simulink model "Model"  (R2018a)
settings: Solver=ode2  StartTime=0.0  StopTime=inf  FixedStep=Ts  RelTol=1e-3
PreLoadFcn:
  | k_synchronize=2;
InitFcn:
  | k_synchronize=2;
  | lego_drive_closedloop_InitData.mdl = get_param(bdroot,'Name');
  | lego_drive_closedloop_InitData.cs = getActiveConfigSet(lego_drive_closedloop_InitData.mdl);
values from neighbouring files (symbols this model uses):
  AxeLength = 31    [robotParam.m]
  D_DeadBand = 2    [robotParam.m]
  EncRes = 2048    [robotParam.m]
  RateLimitHigh = 10    [robotParam.m]
  RateLimitLow = -30    [robotParam.m]
  theta0 = 0    [robotParam.m]
  WheelRadius = 2    [robotParam.m]
  x0 = 0    [robotParam.m]
  y0 = 0    [robotParam.m]
libraries: arduinolib x6, simulink x3, simulink_extras x1
CloseFcn:
  | clear k_synchronize lego_drive_closedloop_InitData
settings Model: SimulationMode=external  ExtModeTrigDuration=2  Creator=The MathWorks, Inc.  LastModifiedBy=root
settings DataIOCC: LimitDataPoints=on  SaveFormat=Array
settings OptimizationCC: ExpressionDepthLimit=2147483647  LifeSpan=Inf  MaxStackSize=64
settings DebuggingCC: UnderspecifiedInitializationDetection=Classic  MergeDetectMultiDrivingBlocksExec=none  InheritedTsInSrcMsg=none  ParameterPrecisionLossMsg=none  FcnCallInpInsideContextMsg=warning  AllowSymbolicDim=off  StateNameClashWarn=warning  SFUnexpectedBacktrackingDiag=warning  SFNoUnconditionalDefaultTransitionDiag=warning  SFExecutionAtInitializationDiag=none
settings HardwareCC: ProdBitPerInt=16  ProdBitPerPointer=16  ProdBitPerSizeT=16  ProdBitPerPtrDiffT=16  ProdLargestAtomicFloat=None  ProdWordSize=8  ProdHWDeviceType=Atmel->AVR  UseEmbeddedCoderFeatures=off  UseSimulinkCoderFeatures=off
settings ModelReferenceCC: PropagateSignalLabelsOutOfModel=off
settings SFSimCC: MATLABDynamicMemAlloc=off
settings RTWCC: SystemTargetFile=ert.tlc  HardwareBoard=Arduino Mega 2560  TemplateMakefile=ert_default_tmf  GenerateReport=on  RTWVerbose=off  Toolchain=Arduino AVR  BuildConfiguration=Faster Runs  LaunchReport=on
settings CodeAppCC: ForceParamTrailComments=on  OperatorAnnotations=on  MangleLength=10  StateflowObjectComments=on  MATLABSourceComments=on
settings ERTTargetCC: MultiwordLength=2048  ERTCustomFileBanners=off  SupportContinuousTime=on  SupportNonInlinedSFcns=on  RemoveResetFunc=off  ModelStepFunctionPrototypeControlCompliant=off
settings ConfigComp: CovMetricSettings=dw  CovHtmlReporting=on  CovSaveCumulativeToWorkspaceVar=on  CovSaveSingleToWorkspaceVar=on  CovExternalEMLEnable=off  CovSFcnEnable=off

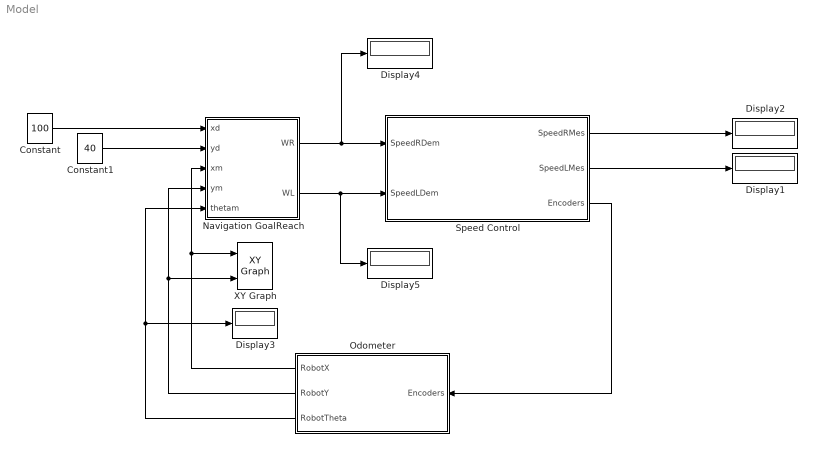
== system Model ==
  Constant : Constant  Value=100
  Constant1 : Constant  Value=40
  Display{1..5} (5 alike) : Display
  Navigation GoalReach : Subsystem
  Odometer : Subsystem
  Speed Control : Subsystem
  XY Graph : simulink/Sinks/XY Graph  xmin=-50  xmax=120  ymin=-50  ymax=120  st=-1
  wires:
  Navigation GoalReach/1(WR) -> Display4/1, Speed Control/1(SpeedRDem)
  Navigation GoalReach/2(WL) -> Display5/1, Speed Control/2(SpeedLDem)
  Speed Control/2(SpeedLMes) -> Display1/1
  Odometer/1(RobotX) -> XY Graph/1, Navigation GoalReach/3(xm)
  Odometer/2(RobotY) -> XY Graph/2, Navigation GoalReach/4(ym)
  Odometer/3(RobotTheta) -> Display3/1, Navigation GoalReach/5(thetam)
  Constant/1 -> Navigation GoalReach/1(xd)
  Constant1/1 -> Navigation GoalReach/2(yd)
  Speed Control/1(SpeedRMes) -> Display2/1
  Speed Control/3(Encoders) -> Odometer/1(Encoders)

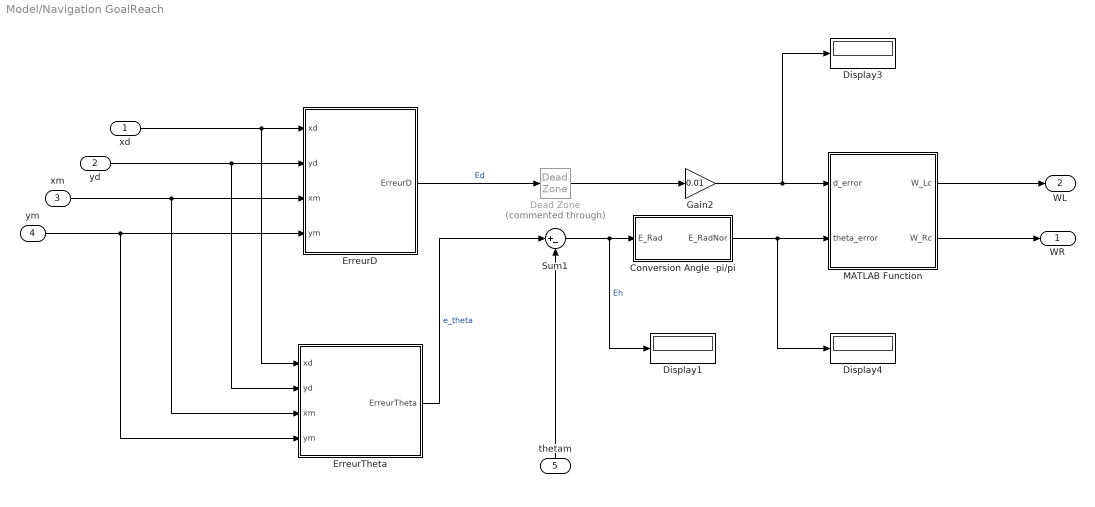
== system Model/Navigation GoalReach ==
  xd : Inport
  yd : Inport  Port=2
  xm : Inport  Port=3
  ym : Inport  Port=4
  thetam : Inport  Port=5
  Conversion Angle -pi/pi : Subsystem
  Dead Zone : DeadZone  Commented=through  LowerValue=-D_DeadBand  UpperValue=D_DeadBand  SaturateOnIntegerOverflow=on
  Display1 : Display
  Display3 : Display
  Display4 : Display
  ErreurD : Subsystem
  ErreurTheta : Subsystem
  Gain2 : Gain  Gain=0.01
  MATLAB Function : MATLAB Function  TreatAsAtomicUnit=on
  Sum1 : Sum  Inputs=|+-
  WR : Outport
  WL : Outport  Port=2
  wires:
  ErreurTheta/1(ErreurTheta) -> Sum1/1  "e_theta"
  xm/1 -> ErreurTheta/3(xm), ErreurD/3(xm)
  ym/1 -> ErreurTheta/4(ym), ErreurD/4("ym ")
  ErreurD/1(ErreurD) -> Dead Zone/1  "Ed"
  Sum1/1 -> Conversion Angle -pi/pi/1("E_Rad "), Display1/1  "Eh"
  thetam/1 -> Sum1/2
  xd/1 -> ErreurTheta/1(xd), ErreurD/1(xd)
  yd/1 -> ErreurTheta/2(yd), ErreurD/2(yd)
  Gain2/1 -> Display3/1, MATLAB Function/1(d_error)
  Conversion Angle -pi/pi/1(E_RadNor) -> Display4/1, MATLAB Function/2(theta_error)
  Dead Zone/1 -> Gain2/1
  MATLAB Function/1(W_Lc) -> WL/1
  MATLAB Function/2(W_Rc) -> WR/1

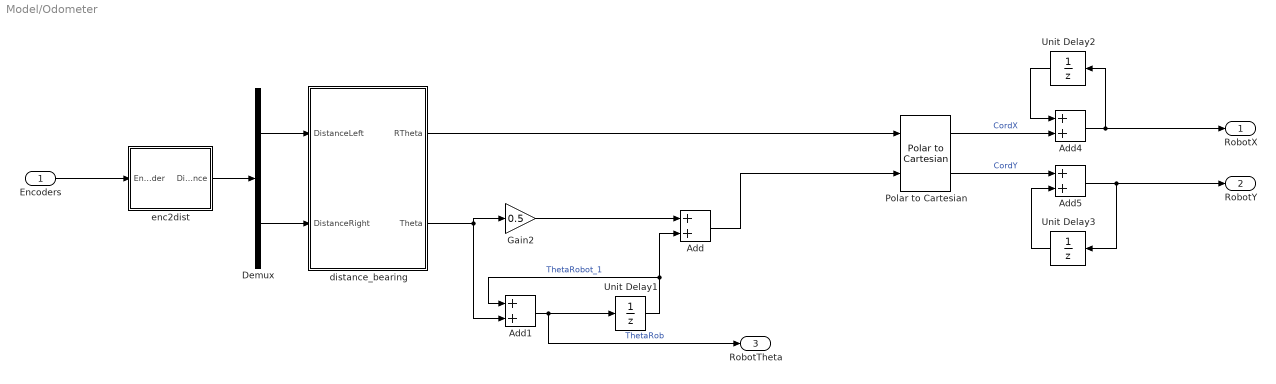
== system Model/Odometer ==
  Encoders : Inport
  Add{,1,4..5} (4 alike) : Sum
  Demux : Demux  Outputs=2
  Gain2 : Gain  Gain=0.5
  Polar to Cartesian : simulink_extras/Transformations/Polar to Cartesian
      settings: SourceProductName=Simulink  SourceProductBaseCode=SL
  Unit Delay1 : UnitDelay  DialogController=Simulink.DDGSource  InitialCondition=theta0*pi/180  SampleTime=-1
  Unit Delay2 : UnitDelay  DialogController=Simulink.DDGSource  InitialCondition=x0  SampleTime=-1
  Unit Delay3 : UnitDelay  DialogController=Simulink.DDGSource  InitialCondition=y0  SampleTime=-1
  distance_bearing : Subsystem
  enc2dist : Subsystem
  RobotX : Outport
  RobotY : Outport  Port=2
  RobotTheta : Outport  Port=3
  wires:
  Gain2/1 -> Add/1
  Polar to Cartesian/1 -> Add4/2  "CordX"
  Polar to Cartesian/2 -> Add5/1  "CordY"
  Unit Delay2/1 -> Add4/1
  Unit Delay3/1 -> Add5/2
  distance_bearing/2(Theta) -> Gain2/1, Add1/2
  Unit Delay1/1 -> Add1/1, Add/2  "ThetaRobot_1"
  Add/1 -> Polar to Cartesian/2
  Add1/1 -> RobotTheta/1, Unit Delay1/1  "ThetaRob"
  distance_bearing/1(RTheta) -> Polar to Cartesian/1
  Add4/1 -> RobotX/1, Unit Delay2/1
  enc2dist/1(Distance) -> Demux/1
  Demux/1 -> distance_bearing/1(DistanceLeft)
  Demux/2 -> distance_bearing/2(DistanceRight)
  Encoders/1 -> enc2dist/1(Encoder)
  Add5/1 -> RobotY/1, Unit Delay3/1

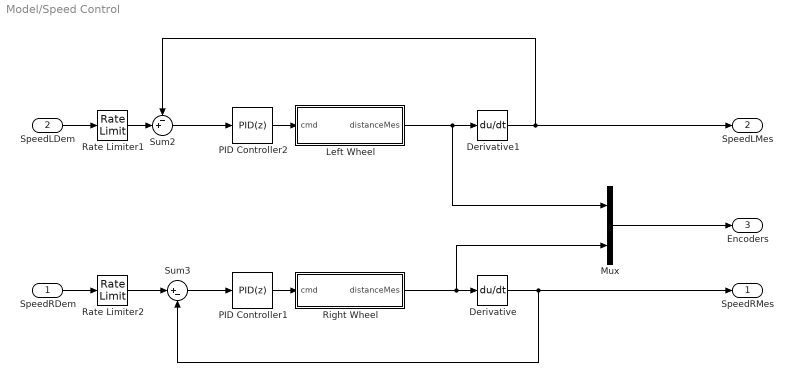
== system Model/Speed Control ==
  SpeedRDem : Inport
  SpeedLDem : Inport  Port=2
  " Left Wheel" : Subsystem
  Derivative : Derivative
  Derivative1 : Derivative
  Mux : Mux  Inputs=2
  PID Controller1 : simulink/Continuous/PID Controller  Controller=PID  TimeDomain=Discrete-time  SampleTime=-1  IntegratorMethod=Forward Euler  FilterMethod=Forward Euler  Form=Parallel  UseFilter=off  ControllerParametersSource=internal  P=0.030  I=0.001  D=0  N=1  InitialConditionSource=internal  InitialConditionForIntegrator=0  InitialConditionForFilter=0  ExternalReset=none  LimitOutput=on  UpperSaturationLimit=1  LowerSaturationLimit=-1  LinearizeAsGain=on  AntiWindupMode=clamping  Kb=1  TrackingMode=off  Kt=1  PParamMin=[]  PParamMax=[]  IParamMin=[]  IParamMax=[]  DParamMin=[]  DParamMax=[]  NParamMin=[]  NParamMax=[]  KbParamMin=[]  KbParamMax=[]  KtParamMin=[]  KtParamMax=[]  POutMin=[]  POutMax=[]  IOutMin=[]  IOutMax=[]  DOutMin=[]  DOutMax=[]  NOutMin=[]  NOutMax=[]  KbOutMin=[]  KbOutMax=[]  KtOutMin=[]  KtOutMax=[]  IntegratorOutMin=[]  IntegratorOutMax=[]  FilterOutMin=[]  FilterOutMax=[]  SumOutMin=[]  SumOutMax=[]  SumI1OutMin=[]  SumI1OutMax=[]  SumI2OutMin=[]  SumI2OutMax=[]  SumI3OutMin=[]  SumI3OutMax=[]  SumDOutMin=[]  SumDOutMax=[]  SaturationOutMin=[]  SaturationOutMax=[]  IntegratorContinuousStateAttributes=''  IntegratorStateMustResolveToSignalObject=off  IntegratorRTWStateStorageClass=Auto  FilterContinuousStateAttributes=''  FilterStateMustResolveToSignalObject=off  FilterRTWStateStorageClass=Auto  DifferentiatorICPrevScaledInput=0  DifferentiatorOutMin=[]  DifferentiatorOutMax=[]  FilterDiffOutCoefMin=[]  FilterDiffOutCoefMax=[]  SumDenOutMin=[]  SumDenOutMax=[]  SumNumOutMin=[]  SumNumOutMax=[]  ReciprocalOutMin=[]  ReciprocalOutMax=[]  DivideOutMin=[]  DivideOutMax=[]  TunerSelectOption=Transfer Function Based (PID Tuner App)
  PID Controller2 : simulink/Continuous/PID Controller  Controller=PID  TimeDomain=Discrete-time  SampleTime=-1  IntegratorMethod=Forward Euler  FilterMethod=Forward Euler  Form=Parallel  UseFilter=off  ControllerParametersSource=internal  P=0.020  I=0.001  D=0  N=1  InitialConditionSource=internal  InitialConditionForIntegrator=0  InitialConditionForFilter=0  ExternalReset=none  LimitOutput=on  UpperSaturationLimit=1  LowerSaturationLimit=-1  LinearizeAsGain=on  AntiWindupMode=clamping  Kb=1  TrackingMode=off  Kt=1  PParamMin=[]  PParamMax=[]  IParamMin=[]  IParamMax=[]  DParamMin=[]  DParamMax=[]  NParamMin=[]  NParamMax=[]  KbParamMin=[]  KbParamMax=[]  KtParamMin=[]  KtParamMax=[]  POutMin=[]  POutMax=[]  IOutMin=[]  IOutMax=[]  DOutMin=[]  DOutMax=[]  NOutMin=[]  NOutMax=[]  KbOutMin=[]  KbOutMax=[]  KtOutMin=[]  KtOutMax=[]  IntegratorOutMin=[]  IntegratorOutMax=[]  FilterOutMin=[]  FilterOutMax=[]  SumOutMin=[]  SumOutMax=[]  SumI1OutMin=[]  SumI1OutMax=[]  SumI2OutMin=[]  SumI2OutMax=[]  SumI3OutMin=[]  SumI3OutMax=[]  SumDOutMin=[]  SumDOutMax=[]  SaturationOutMin=[]  SaturationOutMax=[]  IntegratorContinuousStateAttributes=''  IntegratorStateMustResolveToSignalObject=off  IntegratorRTWStateStorageClass=Auto  FilterContinuousStateAttributes=''  FilterStateMustResolveToSignalObject=off  FilterRTWStateStorageClass=Auto  DifferentiatorICPrevScaledInput=0  DifferentiatorOutMin=[]  DifferentiatorOutMax=[]  FilterDiffOutCoefMin=[]  FilterDiffOutCoefMax=[]  SumDenOutMin=[]  SumDenOutMax=[]  SumNumOutMin=[]  SumNumOutMax=[]  ReciprocalOutMin=[]  ReciprocalOutMax=[]  DivideOutMin=[]  DivideOutMax=[]  TunerSelectOption=Transfer Function Based (PID Tuner App)
  Rate Limiter1 : RateLimiter  RisingSlewLimit=RateLimitHigh  FallingSlewLimit=RateLimitLow  SampleTimeMode=inherited
  Rate Limiter2 : RateLimiter  RisingSlewLimit=RateLimitHigh  FallingSlewLimit=RateLimitLow  SampleTimeMode=inherited
  Right Wheel : Subsystem
  Sum2 : Sum  Inputs=-+|
  Sum3 : Sum  Inputs=|+-
  SpeedRMes : Outport
  SpeedLMes : Outport  Port=2
  Encoders : Outport  Port=3
  wires:
  Derivative1/1 -> SpeedLMes/1, Sum2/1
  Derivative/1 -> SpeedRMes/1, Sum3/2
  PID Controller1/1 -> Right Wheel/1(cmd)
  " Left Wheel"/1(distanceMes) -> Mux/1, Derivative1/1
  Sum3/1 -> PID Controller1/1
  Right Wheel/1(distanceMes) -> Mux/2, Derivative/1
  Sum2/1 -> PID Controller2/1
  PID Controller2/1 -> " Left Wheel"/1(cmd)
  SpeedLDem/1 -> Rate Limiter1/1
  Mux/1 -> Encoders/1
  SpeedRDem/1 -> Rate Limiter2/1
  Rate Limiter1/1 -> Sum2/2
  Rate Limiter2/1 -> Sum3/1

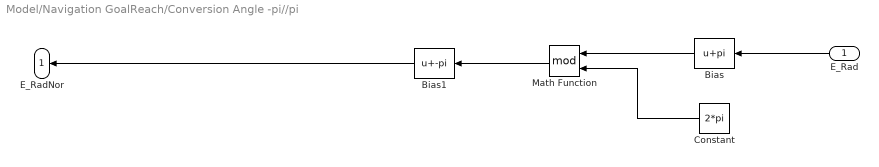
== system Model/Navigation GoalReach/Conversion Angle -pi//pi ==
  "E_Rad " : Inport
  Bias : Bias  Bias=pi
  Bias1 : Bias  Bias=-pi
  Constant : Constant  Value=2*pi  OutDataTypeStr=Inherit: Inherit via back propagation  SampleTime=-1
  Math Function : Math  Operator=mod  SaturateOnIntegerOverflow=on
  E_RadNor : Outport
  wires:
  Bias/1 -> Math Function/1
  Math Function/1 -> Bias1/1
  Constant/1 -> Math Function/2
  Bias1/1 -> E_RadNor/1
  "E_Rad "/1 -> Bias/1

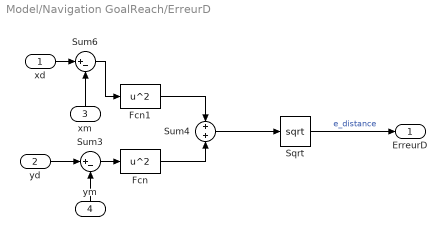
== system Model/Navigation GoalReach/ErreurD ==
  xd : Inport
  yd : Inport  Port=2
  xm : Inport  Port=3
  "ym " : Inport  Port=4
  Fcn : Fcn  Expr=u^2
  Fcn1 : Fcn  Expr=u^2
  Sqrt : Sqrt  SaturateOnIntegerOverflow=on
  Sum3 : Sum  Inputs=|+-
  Sum4 : Sum  Inputs=+|+
  Sum6 : Sum  Inputs=|+-
  ErreurD : Outport
  wires:
  "ym "/1 -> Sum3/2
  xd/1 -> Sum6/1
  xm/1 -> Sum6/2
  yd/1 -> Sum3/1
  Sum6/1 -> Fcn1/1
  Sum3/1 -> Fcn/1
  Fcn1/1 -> Sum4/1
  Sqrt/1 -> ErreurD/1  "e_distance"
  Sum4/1 -> Sqrt/1
  Fcn/1 -> Sum4/2

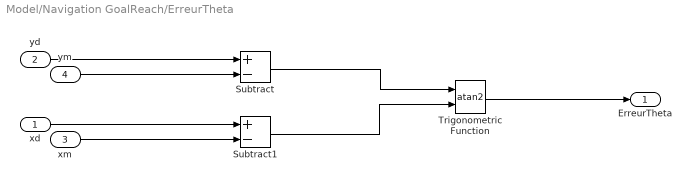
== system Model/Navigation GoalReach/ErreurTheta ==
  xd : Inport
  yd : Inport  Port=2
  xm : Inport  Port=3
  ym : Inport  Port=4
  Subtract : Sum  Inputs=+-
  Subtract1 : Sum  Inputs=+-
  Trigonometric Function : Trigonometry  Operator=atan2  OutputSignalType=real
  ErreurTheta : Outport
  wires:
  xm/1 -> Subtract1/2
  ym/1 -> Subtract/2
  xd/1 -> Subtract1/1
  yd/1 -> Subtract/1
  Trigonometric Function/1 -> ErreurTheta/1
  Subtract/1 -> Trigonometric Function/1
  Subtract1/1 -> Trigonometric Function/2

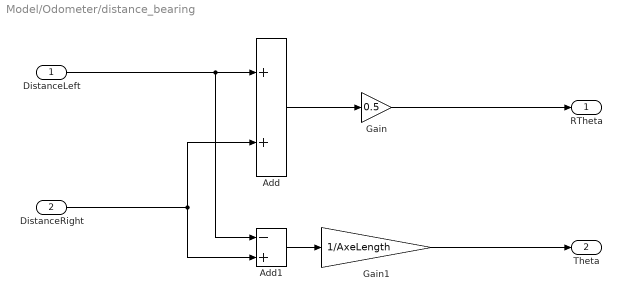
== system Model/Odometer/distance_bearing ==
  DistanceLeft : Inport
  DistanceRight : Inport  Port=2
  Add : Sum
  Add1 : Sum  Inputs=-+
  Gain : Gain  Gain=0.5
  Gain1 : Gain  Gain=1/AxeLength
  RTheta : Outport
  Theta : Outport  Port=2
  wires:
  Gain1/1 -> Theta/1
  Add/1 -> Gain/1
  Gain/1 -> RTheta/1
  Add1/1 -> Gain1/1
  DistanceLeft/1 -> Add1/1, Add/1
  DistanceRight/1 -> Add/2, Add1/2

== system Model/Odometer/enc2dist ==
  Encoder : Inport
  Add2 : Sum  Inputs=-+
  Unit Delay : UnitDelay  DialogController=Simulink.DDGSource  SampleTime=-1
  Distance : Outport
  wires:
  Encoder/1 -> Unit Delay/1, Add2/2
  Unit Delay/1 -> Add2/1
  Add2/1 -> Distance/1

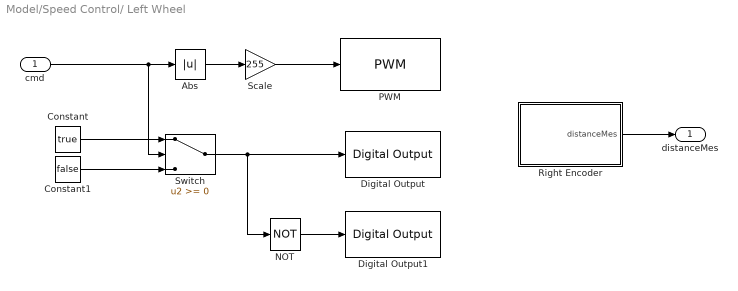
== system Model/Speed Control/ Left Wheel ==
  cmd : Inport
  " Right Encoder " : Subsystem  mask{encoderId=1, CanalAPin=20, CanalBPin=21, Parameter6=0}
      mask prompts: CanalAPin "Encoder Canal A Pin"; CanalBPin "Encoder Canal B Pin"
  Abs : Abs
  Constant : Constant  Value=true  OutDataTypeStr=boolean  SampleTime=-1
  Constant1 : Constant  Value=false  OutDataTypeStr=boolean  SampleTime=-1
  Digital Output : arduinolib/Digital Output  pinNumber=6  blockPlatform=arduino
  Digital Output1 : arduinolib/Digital Output  pinNumber=7  blockPlatform=arduino
  NOT : Logic  Operator=NOT  IconShape=distinctive  AllPortsSameDT=off  OutDataTypeStr=boolean
  PWM : arduinolib/PWM  pinNumber=5  EnableInputFrequency=off  InitialFrequency=2000  InitialDutyCycle=0  NotificationType=None  blockPlatform=arduino
  Scale : Gain  Gain=255
  Switch : Switch
  distanceMes : Outport
  wires:
  " Right Encoder "/1(distanceMes) -> distanceMes/1
  NOT/1 -> Digital Output1/1
  Scale/1 -> PWM/1
  Constant1/1 -> Switch/3
  cmd/1 -> Switch/2, Abs/1
  Constant/1 -> Switch/1
  Abs/1 -> Scale/1
  Switch/1 -> NOT/1, Digital Output/1

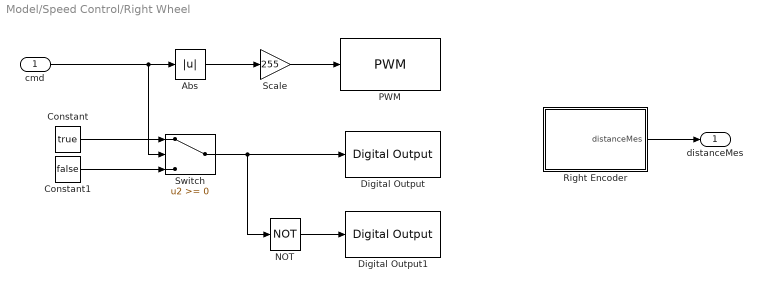
== system Model/Speed Control/Right Wheel ==
  cmd : Inport
  " Right Encoder " : Subsystem  mask{encoderId=0, CanalAPin=19, CanalBPin=18, Parameter6=0}
      mask prompts: CanalAPin "Encoder Canal A Pin"; CanalBPin "Encoder Canal B Pin"
  Abs : Abs
  Constant : Constant  Value=true  OutDataTypeStr=boolean  SampleTime=-1
  Constant1 : Constant  Value=false  OutDataTypeStr=boolean  SampleTime=-1
  Digital Output : arduinolib/Digital Output  pinNumber=4  blockPlatform=arduino
  Digital Output1 : arduinolib/Digital Output  pinNumber=3  blockPlatform=arduino
  NOT : Logic  Operator=NOT  IconShape=distinctive  AllPortsSameDT=off  OutDataTypeStr=boolean
  PWM : arduinolib/PWM  pinNumber=2  EnableInputFrequency=off  InitialFrequency=2000  InitialDutyCycle=0  NotificationType=None  blockPlatform=arduino
  Scale : Gain  Gain=255
  Switch : Switch
  distanceMes : Outport
  wires:
  " Right Encoder "/1(distanceMes) -> distanceMes/1
  NOT/1 -> Digital Output1/1
  Abs/1 -> Scale/1
  Switch/1 -> NOT/1, Digital Output/1
  Scale/1 -> PWM/1
  Constant/1 -> Switch/1
  cmd/1 -> Switch/2, Abs/1
  Constant1/1 -> Switch/3

== system Model/Speed Control/ Left Wheel/ Right Encoder  ==
  Encoder : S-Function  InitFcn=try, set_param(gcb,'FunctionName','sfcn_encoder'), end  FunctionName=sfcn_encoder  Parameters=uint8(encoderId),uint8(CanalAPin),uint8(CanalBPin)  SFunctionModules=sfcn_encoder_wrapper  SFunctionDeploymentMode=off  EnableBusSupport=off  mask(S-Function Builder){}
      mask init:
      | val = [[.9  0.75 0.75 1 1 .9 .9 1]',[1 1 0.75 0.75 .9 .9 1 .9]'];try , sys = get_param(gcb,'SfunBuilderFcnName');if isempty(sys), sys = get_param(gcb,'FunctionName'); end,catch, sys = get_param(gcb,'FunctionName'); end
      settings: CopyFcn=set_param(gcbh,'LinkStatus','none')  PreSaveFcn=try, set_param(gcb,'FunctionName','sfcn_encoder'), end  OpenFcn=sfunctionwizard(gcbh)
      mask Display: plot(val(:,1),val(:,2)),disp(sys), port_label('output',1,'pos')
  Rollover : Subsystem
  divide by time step1 : Gain  Gain=2*pi*WheelRadius/EncRes
  distanceMes : Outport
  wires:
  divide by time step1/1 -> distanceMes/1
  Encoder/1 -> Rollover/1(counts)
  Rollover/1(" mod counts") -> divide by time step1/1

== system Model/Speed Control/Right Wheel/ Right Encoder  ==
  Display : Display
  Encoder : S-Function  InitFcn=try, set_param(gcb,'FunctionName','sfcn_encoder'), end  FunctionName=sfcn_encoder  Parameters=uint8(encoderId),uint8(CanalAPin),uint8(CanalBPin)  SFunctionModules=sfcn_encoder_wrapper  SFunctionDeploymentMode=off  EnableBusSupport=off  mask(S-Function Builder){}
      mask init: same as Model/Speed Control/ Left Wheel/ Right Encoder /Encoder
      settings: CopyFcn=set_param(gcbh,'LinkStatus','none')  PreSaveFcn=try, set_param(gcb,'FunctionName','sfcn_encoder'), end  OpenFcn=sfunctionwizard(gcbh)
      mask Display: plot(val(:,1),val(:,2)),disp(sys), port_label('output',1,'pos')
  Rollover : Subsystem
  divide by time step1 : Gain  Gain=2*pi*WheelRadius/EncRes
  distanceMes : Outport
  wires:
  divide by time step1/1 -> distanceMes/1, Display/1
  Encoder/1 -> Rollover/1(counts)
  Rollover/1(" mod counts") -> divide by time step1/1

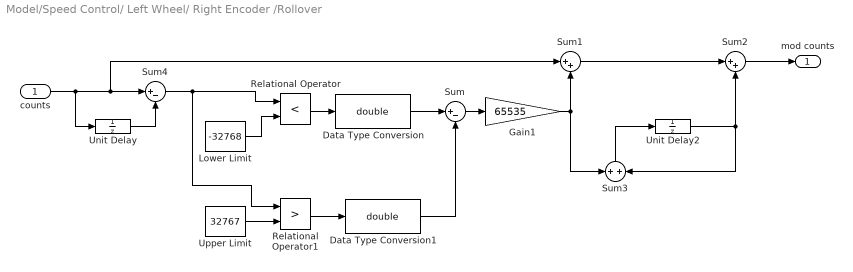
== system Model/Speed Control/ Left Wheel/ Right Encoder /Rollover ==
  counts : Inport
  " Lower Limit" : Constant  Value=-32768
  " Upper Limit" : Constant  Value=32767
  Data Type Conversion : DataTypeConversion  OutDataTypeStr=double  RndMeth=Zero
  Data Type Conversion1 : DataTypeConversion  OutDataTypeStr=double  RndMeth=Zero
  Gain1 : Gain  Gain=65535
  Relational Operator : RelationalOperator  Operator=<  OutDataTypeStr=boolean  RndMeth=Nearest
  Relational Operator1 : RelationalOperator  Operator=>  OutDataTypeStr=boolean  RndMeth=Nearest
  Sum : Sum  Inputs=|+-
  Sum1 : Sum  Inputs=|++
  Sum2 : Sum  Inputs=|++
  Sum3 : Sum
  Sum4 : Sum  Inputs=|+-
  Unit Delay : UnitDelay  SampleTime=-1
  Unit Delay2 : UnitDelay  SampleTime=-1
  " mod counts" : Outport
  wires:
  counts/1 -> Unit Delay/1, Sum1/1, Sum4/1
  Sum2/1 -> " mod counts"/1
  Unit Delay/1 -> Sum4/2
  Data Type Conversion/1 -> Sum/1
  Sum3/1 -> Unit Delay2/1
  Data Type Conversion1/1 -> Sum/2
  Sum/1 -> Gain1/1
  Gain1/1 -> Sum1/2, Sum3/1
  Relational Operator1/1 -> Data Type Conversion1/1
  Sum1/1 -> Sum2/1
  Relational Operator/1 -> Data Type Conversion/1
  " Upper Limit"/1 -> Relational Operator1/2
  Unit Delay2/1 -> Sum3/2, Sum2/2
  " Lower Limit"/1 -> Relational Operator/2
  Sum4/1 -> Relational Operator/1, Relational Operator1/1

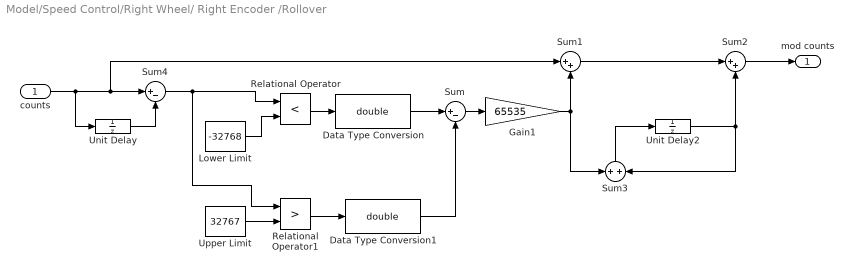
== system Model/Speed Control/Right Wheel/ Right Encoder /Rollover ==
  counts : Inport
  " Lower Limit" : Constant  Value=-32768
  " Upper Limit" : Constant  Value=32767
  Data Type Conversion : DataTypeConversion  OutDataTypeStr=double  RndMeth=Zero
  Data Type Conversion1 : DataTypeConversion  OutDataTypeStr=double  RndMeth=Zero
  Gain1 : Gain  Gain=65535
  Relational Operator : RelationalOperator  Operator=<  OutDataTypeStr=boolean  RndMeth=Nearest
  Relational Operator1 : RelationalOperator  Operator=>  OutDataTypeStr=boolean  RndMeth=Nearest
  Sum : Sum  Inputs=|+-
  Sum1 : Sum  Inputs=|++
  Sum2 : Sum  Inputs=|++
  Sum3 : Sum
  Sum4 : Sum  Inputs=|+-
  Unit Delay : UnitDelay  SampleTime=-1
  Unit Delay2 : UnitDelay  SampleTime=-1
  " mod counts" : Outport
  wires:
  counts/1 -> Unit Delay/1, Sum1/1, Sum4/1
  Sum2/1 -> " mod counts"/1
  Unit Delay/1 -> Sum4/2
  Data Type Conversion/1 -> Sum/1
  Sum3/1 -> Unit Delay2/1
  Data Type Conversion1/1 -> Sum/2
  Sum/1 -> Gain1/1
  Gain1/1 -> Sum1/2, Sum3/1
  Relational Operator1/1 -> Data Type Conversion1/1
  Sum1/1 -> Sum2/1
  Relational Operator/1 -> Data Type Conversion/1
  " Upper Limit"/1 -> Relational Operator1/2
  Unit Delay2/1 -> Sum3/2, Sum2/2
  " Lower Limit"/1 -> Relational Operator/2
  Sum4/1 -> Relational Operator/1, Relational Operator1/1

== matlab function Model/Navigation GoalReach/MATLAB Function ==
  data: d_error input; W_Lc output; theta_error input; W_Rc output
%% Goal_reach fuzzy controller 

function [W_Lc,W_Rc ]= fuzzy_controller_gr(d_error,theta_error)

% fuzzyfication
    D_Z= trianglar_fct( 0.00, 0.08,0 , d_error, 'start');   
    D_NZ= trianglar_fct( 0.03 ,0.15,0.35 , d_error, 'tria');
    D_M= trianglar_fct( 0.25,0.5 ,0.85 , d_error, 'tria');
    D_F= trianglar_fct( 0.70, 1 ,0 , d_error, 'end');
    
    theta_N= trianglar_fct( -45*(pi/180), -15*(pi/180),0 , theta_error, 'start');
    theta_SN= trianglar_fct( -35*(pi/180), -15*(pi/180), -3*(pi/180) , theta_error, 'tria');
    theta_Z= trianglar_fct( -5*(pi/180), 0, 5*(pi/180) , theta_error, 'tria');  % 1 -->1.5
    theta_SP= trianglar_fct( 3*(pi/180), 15*(pi/180), 35*(pi/180) , theta_error, 'tria');
    theta_P= trianglar_fct( 15*(pi/180), 45*(pi/180), 0 , theta_error, 'end');

% activation degree
    Ad=zeros(4,5);
    Ad(1,1)=min([ D_Z theta_N]);
    Ad(1,2)=min([ D_Z theta_SN]);
    Ad(1,3)=min([ D_Z theta_Z]);
    Ad(1,4)=min([ D_Z theta_SP]);
    Ad(1,5)=min([ D_Z theta_P]);
    
    
    Ad(2,1)=min([ D_NZ theta_N]);
    Ad(2,2)=min([ D_NZ theta_SN]);
    Ad(2,3)=min([ D_NZ theta_Z]);
    Ad(2,4)=min([ D_NZ theta_SP]);
    Ad(2,5)=min([ D_NZ theta_P]);
    
    
    Ad(3,1)=min([ D_M theta_N]);
    Ad(3,2)=min([ D_M theta_SN]);
    Ad(3,3)=min([ D_M theta_Z]);
    Ad(3,4)=min([ D_M theta_SP]);
    Ad(3,5)=min([ D_M theta_P]);

    
    Ad(4,1)=min([ D_F theta_N]);
    Ad(4,2)=min([ D_F theta_SN]);
    Ad(4,3)=min([ D_F theta_Z]);
    Ad(4,4)=min([ D_F theta_SP]);
    Ad(4,5)=min([ D_F theta_P]);


 % rules activation
    A_L_Z=  max([ Ad(1,1) Ad(1,2) Ad(1,3) Ad(1,4) Ad(4,1) Ad(1,5)]);
    A_L_M=  max([ Ad(2,1) Ad(2,2) Ad(2,3) Ad(3,1) Ad(3,2) Ad(3,3) Ad(4,2)]);
    A_L_H=  max([ Ad(2,4) Ad(2,5) Ad(3,4) Ad(3,5) Ad(4,3) Ad(4,4) Ad(4,5)]);
    
    A_R_Z=  max([ Ad(1,1) Ad(1,2) Ad(1,3) Ad(1,4) Ad(1,5) Ad(4,5)]);
    A_R_M=  max([ Ad(2,3) Ad(2,4) Ad(2,5) Ad(3,3) Ad(3,4) Ad(3,5) Ad(4,4)]);
    A_R_H=  max([ Ad(2,1) Ad(2,2) Ad(3,1) Ad(3,2) Ad(4,1) Ad(4,2) Ad(4,3)]);
    
    
    R_Z=0;
    R_M=20;
    R_H=40;
    
    L_Z= R_Z;
    L_M= R_M;
    L_H= R_H;

    
    W_Rc= (A_L_Z*L_Z + A_L_M*L_M +  A_L_H*L_H )/(A_L_Z+A_L_M+A_L_H); 
    W_Lc= (A_R_Z*R_Z + A_R_M*R_M +  A_R_H*R_H )/(A_R_Z+A_R_M+A_R_H); 

end
